simulink model "fig_final"  (R2023b)
settings: Solver=VariableStepAuto  StartTime=0.0  StopTime=10.0  RelTol=1e-3
model workspace (MAT data in the model file):
  Tt = 1
  d = 1
values from neighbouring files (symbols this model uses):
  b = 0.1    [Simulador.m]    (also in Simulador2.m = 3.95111589331)
  G = 0.000180    (= 0.00018)    [Simulador.m]    (also in Simulador2.m = 72.312302)
  H = 0.014    [Simulador2.m]
  K = 55555    [Simulador.m]    (also in Simulador2.m = 0.25)
  tau = 0.1    [Simulador.m]    (also in Simulador2.m = 0.43)
  Ti = 0.1    [Simulador.m]    (also in Simulador2.m = 0.43)
  x = 0:0.01:31    [Graficos_lux_Dc.m]    (also in bumpless.m = 0:0.01:27.98)
undefined symbols (not defined in the file or in its folder): x_ref
libraries: visiontextngfix x2
settings Model: Creator=rodsc  LastModifiedBy=rodsc

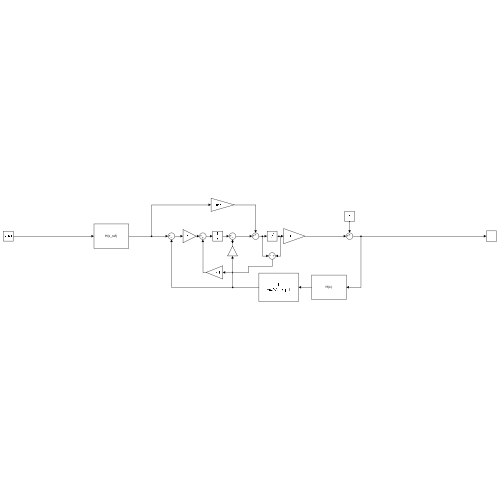
[thumbnail: Simulink's stored preview of the top-level diagram]
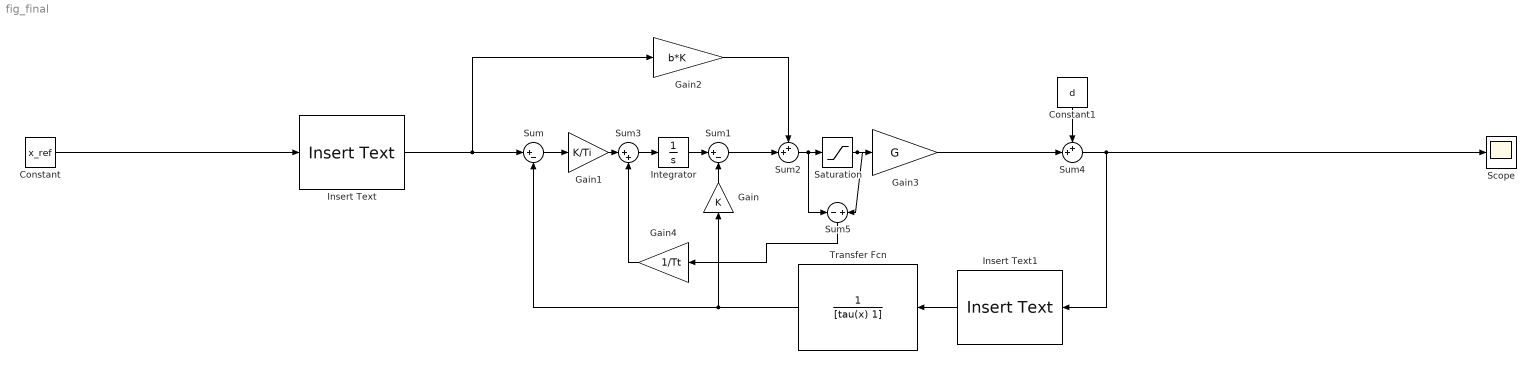
== system fig_final ==
  Constant : Constant  Value=x_ref
  Constant1 : Constant  Value=d
  Gain : Gain  Gain=K
  Gain1 : Gain  Gain=K/Ti
  Gain2 : Gain  Gain=b*K
  Gain3 : Gain  Gain=G
  Gain4 : Gain  Gain=1/Tt
  Insert Text : visiontextngfix/Insert Text  inputType=Obsolete  theText=H(x_ref)  getTextLocFrom=Specify via dialog  textLoc=[1 1]  getTextColorFrom=Specify via dialog  textColor=[0 0 0]  getTextIntensityFrom=Specify via dialog  textIntensity=0  getTextOpacityFrom=Specify via dialog  textOpacity=1.0  dummyVar2=0  dummyVar3=0  dummyVar4=0  imagePorts=One multidimensional signal  isInputTransposed=off  fontFace=LucidaSansRegular  dummyVar1=0  blockFontSize=12  antiAliased=on
  Insert Text1 : visiontextngfix/Insert Text  inputType=Obsolete  theText=H(x)  getTextLocFrom=Specify via dialog  textLoc=[1 1]  getTextColorFrom=Specify via dialog  textColor=[0 0 0]  getTextIntensityFrom=Specify via dialog  textIntensity=0  getTextOpacityFrom=Specify via dialog  textOpacity=1.0  dummyVar2=0  dummyVar3=0  dummyVar4=0  imagePorts=One multidimensional signal  isInputTransposed=off  fontFace=LucidaSansRegular  dummyVar1=0  blockFontSize=12  antiAliased=on
  Integrator : Integrator
  Saturation : Saturate  UpperLimit=4095  LowerLimit=0
  Scope : Scope
  Sum : Sum  Inputs=|+-
  Sum1 : Sum  Inputs=|+-
  Sum2 : Sum  Inputs=++|
  Sum3 : Sum  Inputs=|++
  Sum4 : Sum  Inputs=++|
  Sum5 : Sum  Inputs=-|+
  Transfer Fcn : TransferFcn  Denominator=[tau(x) 1]
  wires:
  Insert Text/1 -> Gain2/1, Sum/1
  Integrator/1 -> Sum1/1
  Sum/1 -> Gain1/1
  Gain/1 -> Sum1/2
  Transfer Fcn/1 -> Gain/1, Sum/2
  Gain3/1 -> Sum4/2
  Sum1/1 -> Sum2/2
  Sum4/1 -> Scope/1, Insert Text1/1
  Constant1/1 -> Sum4/1
  Gain2/1 -> Sum2/1
  Insert Text1/1 -> Transfer Fcn/1
  Constant/1 -> Insert Text/1
  Saturation/1 -> Sum5/2, Gain3/1
  Sum2/1 -> Saturation/1, Sum5/1
  Gain1/1 -> Sum3/1
  Sum3/1 -> Integrator/1
  Gain4/1 -> Sum3/2
  Sum5/1 -> Gain4/1
